simulink model "TST_RWSW"  (Simulink 9.0)
settings: Solver=VariableStepAuto  StartTime=0.0  StopTime=200000  RelTol=1e-3
undefined symbols (not defined in the file or in its folder): ACT_MAG
libraries: DYN x1
settings Model: SuppressorTable=22 serialization::archive 11 0 6 0 0 0 0 0  Creator=WilTravis  LastModifiedBy=WilTravis  SimulationMode=rapid-accelerator
settings DataIOCC: SaveFormat=Dataset
settings OptimizationCC: LifeSpan=auto
settings DebuggingCC: UnderspecifiedInitializationDetection=Simplified  MergeDetectMultiDrivingBlocksExec=error  SFUnexpectedBacktrackingDiag=error  SFNoUnconditionalDefaultTransitionDiag=error  SFExecutionAtInitializationDiag=warning
settings HardwareCC: ProdBitPerPointer=64  ProdBitPerSizeT=64  ProdBitPerPtrDiffT=64  ProdLargestAtomicFloat=Float  ProdIntDivRoundTo=Zero  ProdEndianess=LittleEndian  ProdWordSize=64  ProdHWDeviceType=Intel->x86-64 (Windows64)
settings ModelReferenceCC: PropagateSignalLabelsOutOfModel=on
settings CodeAppCC: StateflowObjectComments=off
settings GRTTargetCC: TargetLangStandard=C99 (ISO)
settings ConfigComp: CovMetricSettings=dwe  CovHtmlReporting=off  CovSaveCumulativeToWorkspaceVar=off  CovSaveSingleToWorkspaceVar=off  CovExternalEMLEnable=on

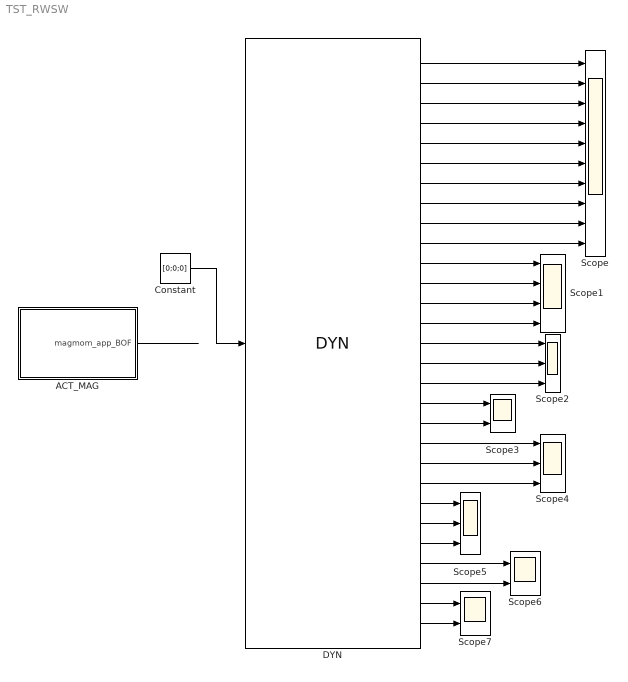
== system TST_RWSW ==
  ACT_MAG : Subsystem
  Constant : Constant  Value=[0;0;0]
  DYN : DYN/DYN
  Scope : Scope  NumInputPorts=10
  Scope1 : Scope  NumInputPorts=4
  Scope2 : Scope  NumInputPorts=3
  Scope3 : Scope  NumInputPorts=2
  Scope4 : Scope  NumInputPorts=3
  Scope5 : Scope  NumInputPorts=3
  Scope6 : Scope  NumInputPorts=2
  Scope7 : Scope  NumInputPorts=2
  wires:
  ACT_MAG/1(magmom_app_BOF) -> ?
  DYN/10 -> Scope/10
  DYN/8 -> Scope/8
  DYN/7 -> Scope/7
  DYN/6 -> Scope/6
  DYN/5 -> Scope/5
  DYN/9 -> Scope/9
  DYN/4 -> Scope/4
  DYN/3 -> Scope/3
  DYN/1 -> Scope/1
  DYN/2 -> Scope/2
  DYN/14 -> Scope1/4
  DYN/13 -> Scope1/3
  DYN/12 -> Scope1/2
  DYN/11 -> Scope1/1
  DYN/17 -> Scope2/3
  DYN/16 -> Scope2/2
  DYN/15 -> Scope2/1
  DYN/19 -> Scope3/2
  DYN/18 -> Scope3/1
  DYN/20 -> Scope4/1
  DYN/21 -> Scope4/2
  DYN/22 -> Scope4/3
  DYN/25 -> Scope5/3
  DYN/24 -> Scope5/2
  DYN/23 -> Scope5/1
  DYN/27 -> Scope6/2
  DYN/26 -> Scope6/1
  DYN/29 -> Scope7/2
  DYN/28 -> Scope7/1
  Constant/1 -> DYN/1

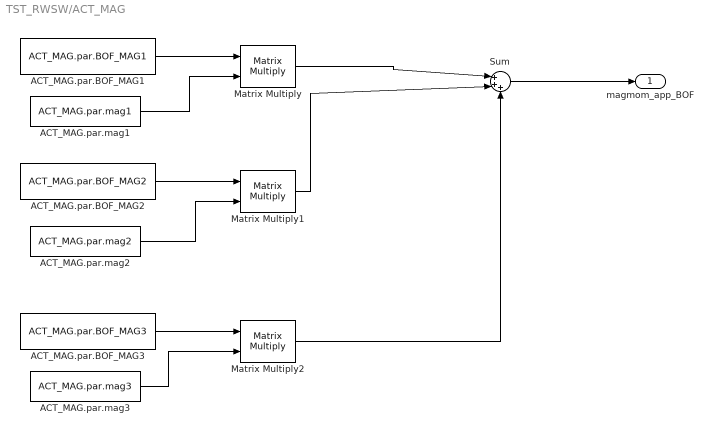
== system TST_RWSW/ACT_MAG ==
  ACT_MAG.par.BOF_MAG1 : Constant  Value=ACT_MAG.par.BOF_MAG1
  ACT_MAG.par.BOF_MAG2 : Constant  Value=ACT_MAG.par.BOF_MAG2
  ACT_MAG.par.BOF_MAG3 : Constant  Value=ACT_MAG.par.BOF_MAG3
  ACT_MAG.par.mag1 : Constant  Value=ACT_MAG.par.mag1
  "ACT_MAG.par.mag2 " : Constant  Value=ACT_MAG.par.mag2
  ACT_MAG.par.mag3 : Constant  Value=ACT_MAG.par.mag3
  Matrix Multiply : Product  Multiplication=Matrix(*)
  Matrix Multiply1 : Product  Multiplication=Matrix(*)
  Matrix Multiply2 : Product  Multiplication=Matrix(*)
  Sum : Sum  Inputs=|+++
  magmom_app_BOF : Outport
  wires:
  Sum/1 -> magmom_app_BOF/1
  Matrix Multiply2/1 -> Sum/3
  Matrix Multiply1/1 -> Sum/2
  Matrix Multiply/1 -> Sum/1
  ACT_MAG.par.BOF_MAG3/1 -> Matrix Multiply2/1
  ACT_MAG.par.mag3/1 -> Matrix Multiply2/2
  ACT_MAG.par.BOF_MAG2/1 -> Matrix Multiply1/1
  "ACT_MAG.par.mag2 "/1 -> Matrix Multiply1/2
  ACT_MAG.par.BOF_MAG1/1 -> Matrix Multiply/1
  ACT_MAG.par.mag1/1 -> Matrix Multiply/2
